simulink model "MotGenEvMapped"  (R2019b)
settings: Solver=FixedStepAuto  StartTime=0.0  StopTime=inf  FixedStep=0.001  RelTol=1e-3  EnableMultiTasking=on
model workspace (MAT data in the model file):
  EV_current = 200
  EV_motion = [20 4 0.8]
  EV_sf = 2000
  Fs = 0
  Fv = 0.0025
  Jcomp = 0.0227
  Ki = 251.3274
  Kisa = 346.6583
  Kp_d = 0.47149
  Kp_q = 0.52125
  Ksa = 85.4316
  Ksf = 1996.2651
  Ld = 0.0003752
  Ldq = [0.0003752 0.0004148]
  Lq = 0.0004148
  Mechanical = [0.0227 0.0025 0]
  P = 4
  PolePairs = 4
  Rs = 0.2
  T_eff_bp = [0 20 40 60 80 100 120 140 160 180 200 220 240 260 280]
  T_max = 120
  T_mtpa = [0 13.3131834767 26.6278836885 39.9456159322 53.2678926341 66.5962219318 79.9321062746 93.277041051 106.632513247 120.000000141]
  Tc = 0.02
  ba = 3.4029
  efficiency_table = [85  85  85  85  85  85  85  85  85  85  85  85  85  85  85; 85  85  85  85  85  85  85  85  85  85  85  85  85  85  85; 85  85  90  90  90  90  90  90  90  90  88  88  88  88  88; 85  85  92  92  92  92  92  92  92  92  92  90  90  90  90; 85  85  92  92  93  93  93  93  92  92  92  90  90  90  90; 85  85  93  94  94  94  94  94  94  94  94  94  94  94  94; 85  85  93  94  94  95  95  95  95  95  95  95  95  95  95; 85  85  93  94  94  95  95  95  95  95  95  95  95  95  95; 85  85  93  94  95  95  95  95  95  95  95  95  95  95  95; 85  85  93  94  95  95  95  95  95  95  95  95  95  95  95; 85  85  93  94  94  94  94  94  94  94  94  94  94  94  94; 85  85  90  92  93  93  93  93  93  93  93  93  93  93  93]
  id_mtpa = [0 -0.114523352646 -0.457989076459 -1.03008464374 -1.83029075221 -2.85788367342 -4.11193850568 -5.59133329791 -7.29475400168 -9.22070020138]
  idq0 = [0 0]
  idq_limits = [-9.220699542 166.993501392 167.247872355]
  iq_mtpa = [0 18.5827440345 37.1633719111 55.7397734896 74.3098506185 92.871523015 111.422734008 129.961456105 148.485696337 166.993501356]
  lambda_pm = 0.1194
  mechanical = [0.0227 0.0025 0]
  omega_init = 0
  power_max = 80000
  theta_init = 0
  torque_max = 280
  w_eff_bp = [0 1000 2000 2728.370453 3000 4000 5000 6000 7000 8000 9000 10000]
libraries: autolibmappedmotor x1
settings Model: ModifiedByFormat=The MathWorks, Inc.  SimulationMode=accelerator  PauseTimes=10  Creator=The MathWorks, Inc.  LastModifiedBy=The MathWorks, Inc.
settings DataIOCC: DSMLogging=off  ReturnWorkspaceOutputs=off
settings DebuggingCC: UnderspecifiedInitializationDetection=Classic  MergeDetectMultiDrivingBlocksExec=none  ArithmeticOperatorsInVariantConditions=warning
settings ModelReferenceCC: PropagateSignalLabelsOutOfModel=off
settings SFSimCC: SimUseLocalCustomCode=off  CustomCodeUndefinedFunction=UseInterfaceOnly
settings RTWCC: RTWUseLocalCustomCode=off
settings CodeAppCC: StateflowObjectComments=on
settings GRTTargetCC: TargetLangStandard=C89/C90 (ANSI)
settings ConfigComp: CovMetricSettings=dsw  CovHtmlReporting=on  CovSaveCumulativeToWorkspaceVar=on  CovSaveSingleToWorkspaceVar=on  CovShowResultsExplorer=off  CovExternalEMLEnable=off
settings SimscapeCC: SimscapeNormalizeSystem=off

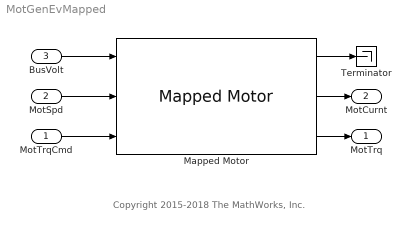
== system MotGenEvMapped ==
  note: Copyright 2015-2018 The MathWorks, Inc.
  MotTrqCmd : Inport
  MotSpd : Inport  Port=2
  BusVolt : Inport  Port=3
  Mapped Motor : autolibmappedmotor/Mapped Motor  port_config=Speed  param_by=Maximum torque and power  w_t=[ 0 375 750 800 ]  T_t=[0.09 0.08 0.07 0]  torque_max=torque_max  power_max=power_max  Tc=Tc  param_loss=Tabulated efficiency data  eff=100  w_eff=375  T_eff=0.08  Piron=0  Pbase=0  w_eff_bp=w_eff_bp.*pi/30  T_eff_bp=T_eff_bp  Temp_eff_bp=[233.15 293.15 373.15]  losses_table=[1 2;3 4]  losses_table_3d=cat(3,[1.49 1.67 2.21 3.10; 0.42 0.69 1.14 2.03; 0.06 0.24 0.78 1.68; 0.42 0.69 1.14 2.03; 1.49 1.67 2.21 3.10],[1.49 1.67 2.21 3.10; 0.42 0.69 1.14 2.03; 0.06 0.24 0.78 1.68; 0.42 0.69 1.14 2.03; 1.49 1.67 2.21 3.10],[1.49 1.67 2.21 3.10; 0.42 0.69 1.14 2.03; 0.06 0.24 0.78 1.68; 0.42 0.69 1.14 2.03; 1.49 1.67 2.21 3.10])  efficiency_table=efficiency_table  efficiency_table_3d=cat(3,[95 95 95 95; 95 95 95 95; 95 95 95 95; 95 95 95 95; 95 95 95 95],[95 95 95 95; 95 95 95 95; 95 95 95 95; 95 95 95 95; 95 95 95 95],[95 95 95 95; 95 95 95 95; 95 95 95 95; 95 95 95 95; 95 95 95 95])  J=5e-6  b=1e-5  omega_o=0  T_t_extended=[0 0.07 0.08 0.09 0.08 0.07 0]  w_t_extended=[-800 -750 -375 0 375 750 800]  KLossIron=0  KLossCopper=0  x_w_eff_vec=[-1047.1975511966 -942.477796076938 -837.758040957278 -733.038285837618 -628.318530717959 -523.598775598299 -418.879020478639 -314.159265358979 -285.714285713875 -209.43951023932 -104.71975511966 0 104.71975511966 209.43951023932 285.714285713875 314.159265358979 418.879020478639 523.598775598299 628.318530717959 733.038285837618 837.758040957278 942.477796076938 1047.1975511966]  x_T_eff_vec=[-280 -260 -240 -220 -200 -180 -160 -140 -120 -100 -80 -60 -40 -20 0 20 40 60 80 100 120 140 160 180 200 220 240 260 280]  x_tmp_eff_vec=[-0.09 -0.06 -0.03 0 0.03 0.06 0.09]  x_losses_mat=[22069.9698961863 20493.5434750302 18917.117053874 17340.6906327178 15764.2642115617 14187.8377904055 12611.4113692493 11034.9849480932 9458.558526937 7882.13210578084 6305.70568462467 5463.63939754746 4654.21133865155 3695.99135716446 0 3141.59265358979 4188.79020478639 5026.54824574367 5864.30628670094 7330.38285837618 8796.45943005141 10262.5360017267 11728.6125734019 13194.6891450771 14660.7657167524 16126.8422884276 17592.9188601028 19058.9954317781 20525.0720034533;16844.2840149921 15641.1208710641 14437.9577271361 13234.7945832081 12031.6314392801 10828.4682953521 9625.30515142405 8422.14200749604 7218.97886356803 6015.81571964003 4812.65257571202 3609.48943178402 2837.5675580811 3326.39222144802 0 2827.43338823081 2638.93782901542 3392.92006587697 4523.8934211693 5654.86677646162 6785.84013175395 7916.81348704627 9047.7868423386 10178.7601976309 11309.7335529232 12440.7069082156 13571.6802635079 14702.6536188002 15833.6269740925;12345.907972002 11464.0574025733 10582.2068331446 9700.35626371584 8818.50569428713 7936.65512485842 7054.8045554297 6172.95398600099 5291.10341657228 4409.25284714356 3527.40227771485 3208.43505047468 2522.28227384987 2956.79308573157 0 2513.27412287184 2345.72251468038 3015.9289474462 3351.03216382911 4188.79020478639 5026.54824574366 5864.30628670094 6702.06432765822 7539.82236861549 8377.58040957277 9215.33845053005 10053.0964914873 10890.8545324446 11728.6125734019;10802.6694755017 10031.0502272516 9259.43097900148 8487.81173075136 7716.19248250124 6944.57323425111 6172.95398600099 5401.33473775087 4629.71548950074 3858.09624125062 3086.47699300049 2807.38066916535 2206.99698961863 2587.19395001512 0 2199.11485751286 2052.50720034533 2638.93782901542 2932.15314335047 3665.19142918809 4398.2297150257 5131.26800086332 5864.30628670094 6597.34457253856 7330.38285837617 8063.42114421379 8796.45943005141 9529.49771588903 10262.5360017266;9259.43097900149 8598.04305192995 7936.65512485842 7275.26719778688 6613.87927071535 5952.49134364381 5291.10341657228 4629.71548950074 3968.32756242921 3306.93963535767 3208.43505047468 2406.32628785601 1891.7117053874 2217.59481429868 0 1884.95559215388 1759.29188601028 2261.94671058465 3015.9289474462 3141.59265358979 3769.91118430775 4398.22971502571 5026.54824574366 5654.86677646162 6283.18530717958 6911.50383789754 7539.82236861549 8168.14089933345 8796.45943005141;7716.19248250124 7165.03587660829 6613.87927071535 6062.7226648224 5511.56605892946 4960.40945303651 4409.25284714356 3858.09624125062 3306.93963535767 2755.78302946473 2673.69587539557 2005.27190654668 1576.42642115617 1847.99567858223 0 1570.7963267949 1466.07657167524 1884.95559215387 2513.27412287183 2617.99387799149 3141.59265358979 3665.19142918809 4188.79020478639 4712.38898038468 5235.98775598298 5759.58653158128 6283.18530717958 6806.78408277788 7330.38285837618;7486.34845110759 6951.60927602848 6416.87010094936 5882.13092587025 5347.39175079114 4812.65257571202 4277.91340063291 3743.17422555379 3208.43505047468 2673.69587539557 2138.95670031645 1604.21752523734 1261.14113692493 1478.39654286579 0 1256.63706143592 1172.86125734019 1507.9644737231 2010.61929829747 2513.27412287183 3015.9289474462 3518.58377202056 4021.23859659493 4523.8934211693 5026.54824574366 5529.20307031803 6031.8578948924 6534.51271946676 7037.16754404113;9773.84381116825 9075.71211037052 8377.58040957279 7679.44870877505 5463.63939754746 4917.27545779272 4370.91151803797 3310.49548442795 2837.5675580811 2364.63963173425 1891.7117053874 1639.09181926424 1092.72787950949 1108.79740714934 0 942.477796076938 1005.30964914873 1507.9644737231 1759.29188601028 2199.11485751285 2638.93782901542 3078.760800518 4021.23859659493 4523.8934211693 5026.54824574367 6911.50383789754 7539.8223686155 8168.14089933346 8796.45943005142;8888.88888887612 8253.9682539564 7619.04761903668 6984.12698411695 4968.94409937174 4472.04968943457 3975.15527949739 3478.26086956022 2981.36645962304 2484.47204968587 1987.5776397487 ...(+6498 chars)]  x_losses_mat_3d=[37.8947368421052 25.2631578947368 12.6315789473684 0 12 24 36;18.9473684210526 12.6315789473684 6.3157894736842 0 5.99999999999999 12 18;0 0 0 0 0 0 0;18 12 5.99999999999999 0 6.3157894736842 12.6315789473684 18.9473684210526;36 24 12 0 12.6315789473684 25.2631578947368 37.8947368421052]  CalLossMapData={}  CalLossWithTempMapData={}  aMode=aMode  RefBlkName='autolibmappedmotor/Mapped Motor'
      settings: SourceProductName=Powertrain Blockset  SourceProductBaseCode=PW
  Terminator : Terminator
  MotTrq : Outport  VectorParamsAs1DForOutWhenUnconnected=off
  MotCurnt : Outport  Port=2  VectorParamsAs1DForOutWhenUnconnected=off
  wires:
  MotTrqCmd/1 -> Mapped Motor/3
  BusVolt/1 -> Mapped Motor/1
  MotSpd/1 -> Mapped Motor/2
  Mapped Motor/3 -> MotTrq/1
  Mapped Motor/2 -> MotCurnt/1
  Mapped Motor/1 -> Terminator/1
